simulink model "subsystem"  (Simulink 7.7)
settings: Solver=ode45  StartTime=0.0  StopTime=10.0  RelTol=1e-3
values from neighbouring files (symbols this model uses):
  k1 = 1/yl    (= 2.5)    [Laboratorio2.m]
  k2 = sqrt(2*k1)    [Laboratorio2.m]
  yl = 0.4    [Laboratorio2.m]
settings Model: Creator=g  LastModifiedBy=g

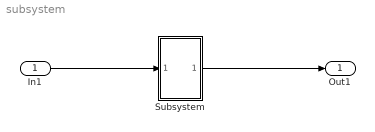
== system subsystem ==
  In1 : Inport
  Subsystem : Subsystem
  Out1 : Outport
  wires:
  Subsystem/1(Out1) -> Out1/1
  In1/1 -> Subsystem/1(In1)

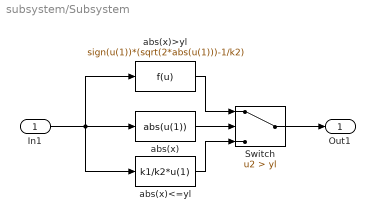
== system subsystem/Subsystem ==
  In1 : Inport
  Switch : Switch  Criteria=u2 > Threshold  Threshold=yl
  abs(x) : Fcn  Expr=abs(u(1))
  abs(x)<=yl : Fcn  Expr=k1/k2*u(1)
  abs(x)>yl : Fcn  Expr=sign(u(1))*(sqrt(2*abs(u(1)))-1/k2)
  Out1 : Outport
  wires:
  In1/1 -> abs(x)>yl/1, abs(x)<=yl/1, abs(x)/1
  abs(x)>yl/1 -> Switch/1
  abs(x)<=yl/1 -> Switch/3
  Switch/1 -> Out1/1
  abs(x)/1 -> Switch/2
